simulink library "halout"  (R2021b)
settings: Solver=VariableStepAuto  StartTime=0.0  StopTime=10.0  RelTol=1e-3
undefined symbols (not defined in the file): C_TASK_5MS_S, FALSE, KHAL_CAN1TxReq_flg, KHAL_CAN2TxReq_flg, KHAL_CAN3FD3VCU1toNIDECTxReq_flg, KHAL_CAN3FD3VCU1TxReq_flg, KHAL_CAN3FD3VCU2E2E_flg, KHAL_CAN3FD3VCU2toNIDECE2E_flg, KHAL_CAN3FD3VCU2toNIDECTxReq_flg, KHAL_CAN3FD3VCU2TxReq_flg, KHAL_CAN3TxReq_flg, KHAL_CAN4FD4CE1000E2E_flg, KHAL_CAN4FD4CE1000TxReq_flg, KHAL_CAN4TxReq_flg, KHAL_CAN5TxReq_flg, KHAL_CAN7TxReq_flg, ONE_INT, TRUE, ZERO_INT
libraries: FVT_lib x258, simulink x115
(part 15 of 17)

== system halout/HAL_OUT/CAN4/FD4_CE100_0_0x116/HornCtrl ==
  HornCtrl : Inport
  Data Type Conversion : DataTypeConversion  OutDataTypeStr=uint8  RndMeth=Round
  CAN4_HornCtrl : Outport
  wires:
  Data Type Conversion/1 -> CAN4_HornCtrl/1
  HornCtrl/1 -> Data Type Conversion/1

== system halout/HAL_OUT/CAN4/FD4_CE100_0_0x116/LAPMWdwEnable ==
  LAPMWdwEnable : Inport
  Data Type Conversion : DataTypeConversion  OutDataTypeStr=uint8  RndMeth=Round
  CAN4_L_APM_WdwEnable : Outport
  wires:
  Data Type Conversion/1 -> CAN4_L_APM_WdwEnable/1
  LAPMWdwEnable/1 -> Data Type Conversion/1

== system halout/HAL_OUT/CAN4/FD4_CE100_0_0x116/LBSD ==
  LBSD : Inport
  Data Type Conversion : DataTypeConversion  OutDataTypeStr=uint8  RndMeth=Round
  CAN4_LBSD : Outport
  wires:
  Data Type Conversion/1 -> CAN4_LBSD/1
  LBSD/1 -> Data Type Conversion/1

== system halout/HAL_OUT/CAN4/FD4_CE100_0_0x116/LBeam ==
  LBeam : Inport
  Data Type Conversion : DataTypeConversion  OutDataTypeStr=uint8  RndMeth=Round
  CAN4_L_Beam : Outport
  wires:
  Data Type Conversion/1 -> CAN4_L_Beam/1
  LBeam/1 -> Data Type Conversion/1

== system halout/HAL_OUT/CAN4/FD4_CE100_0_0x116/LDRL ==
  LDRL : Inport
  Data Type Conversion : DataTypeConversion  OutDataTypeStr=uint8  RndMeth=Round
  CAN4_LDRL : Outport
  wires:
  Data Type Conversion/1 -> CAN4_LDRL/1
  LDRL/1 -> Data Type Conversion/1

== system halout/HAL_OUT/CAN4/FD4_CE100_0_0x116/LTurnLP ==
  LTurnLP : Inport
  Data Type Conversion : DataTypeConversion  OutDataTypeStr=uint8  RndMeth=Round
  CAN4_LTurnLP : Outport
  wires:
  Data Type Conversion/1 -> CAN4_LTurnLP/1
  LTurnLP/1 -> Data Type Conversion/1

== system halout/HAL_OUT/CAN4/FD4_CE100_0_0x116/LampPwr ==
  LampPwr : Inport
  Data Type Conversion : DataTypeConversion  OutDataTypeStr=uint8  RndMeth=Round
  CAN4_LampPwr : Outport
  wires:
  Data Type Conversion/1 -> CAN4_LampPwr/1
  LampPwr/1 -> Data Type Conversion/1

== system halout/HAL_OUT/CAN4/FD4_CE100_0_0x116/LockSetting ==
  LockSetting : Inport
  Data Type Conversion : DataTypeConversion  OutDataTypeStr=uint8  RndMeth=Round
  CAN4_LockSetting : Outport
  wires:
  Data Type Conversion/1 -> CAN4_LockSetting/1
  LockSetting/1 -> Data Type Conversion/1

== system halout/HAL_OUT/CAN4/FD4_CE100_0_0x116/MSACrlSta ==
  MSACrlSta : Inport
  Data Type Conversion : DataTypeConversion  OutDataTypeStr=uint8  RndMeth=Round
  CAN4_MSA_Crl_Sta : Outport
  wires:
  Data Type Conversion/1 -> CAN4_MSA_Crl_Sta/1
  MSACrlSta/1 -> Data Type Conversion/1

== system halout/HAL_OUT/CAN4/FD4_CE100_0_0x116/MirrorCtrl ==
  MirrorCtrl : Inport
  Data Type Conversion : DataTypeConversion  OutDataTypeStr=uint8  RndMeth=Round
  CAN4_MirrorCtrl : Outport
  wires:
  Data Type Conversion/1 -> CAN4_MirrorCtrl/1
  MirrorCtrl/1 -> Data Type Conversion/1

== system halout/HAL_OUT/CAN4/FD4_CE100_0_0x116/MirrorDefog ==
  MirrorDefog : Inport
  Data Type Conversion : DataTypeConversion  OutDataTypeStr=uint8  RndMeth=Round
  CAN4_MirrorDefog : Outport
  wires:
  Data Type Conversion/1 -> CAN4_MirrorDefog/1
  MirrorDefog/1 -> Data Type Conversion/1

== system halout/HAL_OUT/CAN4/FD4_CE100_0_0x116/PosLamp ==
  PosLamp : Inport
  Data Type Conversion : DataTypeConversion  OutDataTypeStr=uint8  RndMeth=Round
  CAN4_PosLamp : Outport
  wires:
  Data Type Conversion/1 -> CAN4_PosLamp/1
  PosLamp/1 -> Data Type Conversion/1

== system halout/HAL_OUT/CAN4/FD4_CE100_0_0x116/PsDoorSW ==
  PsDoorSW : Inport
  Data Type Conversion : DataTypeConversion  OutDataTypeStr=uint8  RndMeth=Round
  CAN4_PsDoorSW : Outport
  wires:
  Data Type Conversion/1 -> CAN4_PsDoorSW/1
  PsDoorSW/1 -> Data Type Conversion/1

== system halout/HAL_OUT/CAN4/FD4_CE100_0_0x116/PwrSta ==
  PwrSta : Inport
  Data Type Conversion : DataTypeConversion  OutDataTypeStr=uint8  RndMeth=Round
  CAN4_PwrSta : Outport
  wires:
  Data Type Conversion/1 -> CAN4_PwrSta/1
  PwrSta/1 -> Data Type Conversion/1

== system halout/HAL_OUT/CAN4/FD4_CE100_0_0x116/RBSD ==
  RBSD : Inport
  Data Type Conversion : DataTypeConversion  OutDataTypeStr=uint8  RndMeth=Round
  CAN4_RBSD : Outport
  wires:
  Data Type Conversion/1 -> CAN4_RBSD/1
  RBSD/1 -> Data Type Conversion/1

== system halout/HAL_OUT/CAN4/FD4_CE100_0_0x116/RCVCU1CAN4 ==
  RCVCU1CAN4 : Inport
  Data Type Conversion : DataTypeConversion  OutDataTypeStr=uint8  RndMeth=Round
  CAN4_RC_VCU1_CAN4 : Outport
  wires:
  Data Type Conversion/1 -> CAN4_RC_VCU1_CAN4/1
  RCVCU1CAN4/1 -> Data Type Conversion/1

== system halout/HAL_OUT/CAN4/FD4_CE100_0_0x116/RDRL ==
  RDRL : Inport
  Data Type Conversion : DataTypeConversion  OutDataTypeStr=uint8  RndMeth=Round
  CAN4_RDRL : Outport
  wires:
  Data Type Conversion/1 -> CAN4_RDRL/1
  RDRL/1 -> Data Type Conversion/1

== system halout/HAL_OUT/CAN4/FD4_CE100_0_0x116/RLDoorSW ==
  RLDoorSW : Inport
  Data Type Conversion : DataTypeConversion  OutDataTypeStr=uint8  RndMeth=Round
  CAN4_RLDoorSW : Outport
  wires:
  Data Type Conversion/1 -> CAN4_RLDoorSW/1
  RLDoorSW/1 -> Data Type Conversion/1

== system halout/HAL_OUT/CAN4/FD4_CE100_0_0x116/RRDoorSW ==
  RRDoorSW : Inport
  Data Type Conversion : DataTypeConversion  OutDataTypeStr=uint8  RndMeth=Round
  CAN4_RRDoorSW : Outport
  wires:
  Data Type Conversion/1 -> CAN4_RRDoorSW/1
  RRDoorSW/1 -> Data Type Conversion/1

== system halout/HAL_OUT/CAN4/FD4_CE100_0_0x116/RTurnLP ==
  RTurnLP : Inport
  Data Type Conversion : DataTypeConversion  OutDataTypeStr=uint8  RndMeth=Round
  CAN4_RTurnLP : Outport
  wires:
  Data Type Conversion/1 -> CAN4_RTurnLP/1
  RTurnLP/1 -> Data Type Conversion/1

== system halout/HAL_OUT/CAN4/FD4_CE100_0_0x116/ReBrakeLPReq ==
  ReBrakeLPReq : Inport
  Data Type Conversion : DataTypeConversion  OutDataTypeStr=uint8  RndMeth=Round
  CAN4_ReBrakeLPReq : Outport
  wires:
  Data Type Conversion/1 -> CAN4_ReBrakeLPReq/1
  ReBrakeLPReq/1 -> Data Type Conversion/1

== system halout/HAL_OUT/CAN4/FD4_CE100_0_0x116/ReverseLamp ==
  ReverseLamp : Inport
  Data Type Conversion : DataTypeConversion  OutDataTypeStr=uint8  RndMeth=Round
  CAN4_ReverseLamp : Outport
  wires:
  Data Type Conversion/1 -> CAN4_ReverseLamp/1
  ReverseLamp/1 -> Data Type Conversion/1

== system halout/HAL_OUT/CAN4/FD4_CE100_0_0x116/RoomLampH ==
  RoomLampH : Inport
  Data Type Conversion : DataTypeConversion  OutDataTypeStr=uint8  RndMeth=Round
  CAN4_RoomLampH : Outport
  wires:
  Data Type Conversion/1 -> CAN4_RoomLampH/1
  RoomLampH/1 -> Data Type Conversion/1

== system halout/HAL_OUT/CAN4/FD4_CE100_0_0x116/RoomLampL ==
  RoomLampL : Inport
  Data Type Conversion : DataTypeConversion  OutDataTypeStr=uint8  RndMeth=Round
  CAN4_RoomLampL : Outport
  wires:
  Data Type Conversion/1 -> CAN4_RoomLampL/1
  RoomLampL/1 -> Data Type Conversion/1

== system halout/HAL_OUT/CAN4/FD4_CE100_0_0x116/RrChargingDoorCtrl ==
  RrChargingDoorCtrl : Inport
  Data Type Conversion : DataTypeConversion  OutDataTypeStr=uint8  RndMeth=Round
  CAN4_Rr_ChargingDoorCtrl : Outport
  wires:
  Data Type Conversion/1 -> CAN4_Rr_ChargingDoorCtrl/1
  RrChargingDoorCtrl/1 -> Data Type Conversion/1

== system halout/HAL_OUT/CAN4/FD4_CE100_0_0x116/RrDefog ==
  RrDefog : Inport
  Data Type Conversion : DataTypeConversion  OutDataTypeStr=uint8  RndMeth=Round
  CAN4_Rr_Defog : Outport
  wires:
  Data Type Conversion/1 -> CAN4_Rr_Defog/1
  RrDefog/1 -> Data Type Conversion/1

== system halout/HAL_OUT/CAN4/FD4_CE100_0_0x116/RrFogLamp ==
  RrFogLamp : Inport
  Data Type Conversion : DataTypeConversion  OutDataTypeStr=uint8  RndMeth=Round
  CAN4_Rr_FogLamp : Outport
  wires:
  Data Type Conversion/1 -> CAN4_Rr_FogLamp/1
  RrFogLamp/1 -> Data Type Conversion/1

== system halout/HAL_OUT/CAN4/FD4_CE100_0_0x116/RrWiper ==
  RrWiper : Inport
  Data Type Conversion : DataTypeConversion  OutDataTypeStr=uint8  RndMeth=Round
  CAN4_Rr_Wiper : Outport
  wires:
  Data Type Conversion/1 -> CAN4_Rr_Wiper/1
  RrWiper/1 -> Data Type Conversion/1

== system halout/HAL_OUT/CAN4/FD4_CE100_0_0x116/ShiftGearPosn ==
  ShiftGearPosn : Inport
  Data Type Conversion : DataTypeConversion  OutDataTypeStr=uint8  RndMeth=Round
  CAN4_ShiftGearPosn : Outport
  wires:
  Data Type Conversion/1 -> CAN4_ShiftGearPosn/1
  ShiftGearPosn/1 -> Data Type Conversion/1

== system halout/HAL_OUT/CAN4/FD4_CE100_0_0x116/TailgateHDSW ==
  TailgateHDSW : Inport
  Data Type Conversion : DataTypeConversion  OutDataTypeStr=uint8  RndMeth=Round
  CAN4_TailgateHDSW : Outport
  wires:
  Data Type Conversion/1 -> CAN4_TailgateHDSW/1
  TailgateHDSW/1 -> Data Type Conversion/1

== system halout/HAL_OUT/CAN4/FD4_CE100_0_0x116/TailgateRemote ==
  TailgateRemote : Inport
  Data Type Conversion : DataTypeConversion  OutDataTypeStr=uint8  RndMeth=Round
  CAN4_TailgateRemote : Outport
  wires:
  Data Type Conversion/1 -> CAN4_TailgateRemote/1
  TailgateRemote/1 -> Data Type Conversion/1

== system halout/HAL_OUT/CAN4/FD4_CE100_0_0x116/TailgateSW ==
  TailgateSW : Inport
  Data Type Conversion : DataTypeConversion  OutDataTypeStr=uint8  RndMeth=Round
  CAN4_Tailgate_SW : Outport
  wires:
  Data Type Conversion/1 -> CAN4_Tailgate_SW/1
  TailgateSW/1 -> Data Type Conversion/1

== system halout/HAL_OUT/CAN4/FD4_CE100_0_0x116/TimeSNDKCFbk ==
  TimeSNDKCFbk : Inport
  Data Type Conversion : DataTypeConversion  OutDataTypeStr=uint32  RndMeth=Round
  CAN4_TimeSNDKCFbk : Outport
  wires:
  Data Type Conversion/1 -> CAN4_TimeSNDKCFbk/1
  TimeSNDKCFbk/1 -> Data Type Conversion/1

== system halout/HAL_OUT/CAN4/FD4_CE100_0_0x116/TrunkRel ==
  TrunkRel : Inport
  Data Type Conversion : DataTypeConversion  OutDataTypeStr=uint8  RndMeth=Round
  CAN4_TrunkRel : Outport
  wires:
  Data Type Conversion/1 -> CAN4_TrunkRel/1
  TrunkRel/1 -> Data Type Conversion/1

== system halout/HAL_OUT/CAN4/FD4_CE100_0_0x116/WasherCtrl ==
  WasherCtrl : Inport
  Data Type Conversion : DataTypeConversion  OutDataTypeStr=uint8  RndMeth=Round
  CAN4_WasherCtrl : Outport
  wires:
  Data Type Conversion/1 -> CAN4_WasherCtrl/1
  WasherCtrl/1 -> Data Type Conversion/1

== system halout/HAL_OUT/CAN4/FD4_CE100_0_0x116/WiperFixMode ==
  WiperFixMode : Inport
  Data Type Conversion : DataTypeConversion  OutDataTypeStr=uint8  RndMeth=Round
  CAN4_WiperFixMode : Outport
  wires:
  Data Type Conversion/1 -> CAN4_WiperFixMode/1
  WiperFixMode/1 -> Data Type Conversion/1

== system halout/HAL_OUT/CAN4/FD4_CE100_1_0x182/ACSubMode ==
  ACSubMode : Inport
  Data Type Conversion : DataTypeConversion  OutDataTypeStr=uint8  RndMeth=Round
  CAN4_ACSubMode : Outport
  wires:
  Data Type Conversion/1 -> CAN4_ACSubMode/1
  ACSubMode/1 -> Data Type Conversion/1

== system halout/HAL_OUT/CAN4/FD4_CE100_1_0x182/APTCActFrRiPwr ==
  APTCActFrRiPwr : Inport
  Data Type Conversion : DataTypeConversion  OutDataTypeStr=uint8  RndMeth=Round
  convert_out : FVT_lib/hal/convert_out  gain=25  offset=0
  CAN4_APTC_ActFrRiPwr : Outport
  wires:
  Data Type Conversion/1 -> CAN4_APTC_ActFrRiPwr/1
  convert_out/1 -> Data Type Conversion/1
  APTCActFrRiPwr/1 -> convert_out/1

== system halout/HAL_OUT/CAN4/FD4_CE100_1_0x182/BatLoopActWtFlw ==
  BatLoopActWtFlw : Inport
  Data Type Conversion : DataTypeConversion  OutDataTypeStr=uint8  RndMeth=Round
  convert_out : FVT_lib/hal/convert_out  gain=0.1  offset=-5
  CAN4_BatLoopActWtFlw : Outport
  wires:
  Data Type Conversion/1 -> CAN4_BatLoopActWtFlw/1
  convert_out/1 -> Data Type Conversion/1
  BatLoopActWtFlw/1 -> convert_out/1

== system halout/HAL_OUT/CAN4/FD4_CE100_1_0x182/BatteryMode ==
  BatteryMode : Inport
  Data Type Conversion : DataTypeConversion  OutDataTypeStr=uint8  RndMeth=Round
  CAN4_BatteryMode : Outport
  wires:
  Data Type Conversion/1 -> CAN4_BatteryMode/1
  BatteryMode/1 -> Data Type Conversion/1

== system halout/HAL_OUT/CAN4/FD4_CE100_1_0x182/CCUACLampSts ==
  CCUACLampSts : Inport
  Data Type Conversion : DataTypeConversion  OutDataTypeStr=uint8  RndMeth=Round
  CAN4_CCU_ACLampSts : Outport
  wires:
  Data Type Conversion/1 -> CAN4_CCU_ACLampSts/1
  CCUACLampSts/1 -> Data Type Conversion/1

== system halout/HAL_OUT/CAN4/FD4_CE100_1_0x182/CCUACMaxLampSts ==
  CCUACMaxLampSts : Inport
  Data Type Conversion : DataTypeConversion  OutDataTypeStr=uint8  RndMeth=Round
  CAN4_CCU_ACMaxLampSts : Outport
  wires:
  Data Type Conversion/1 -> CAN4_CCU_ACMaxLampSts/1
  CCUACMaxLampSts/1 -> Data Type Conversion/1

== system halout/HAL_OUT/CAN4/FD4_CE100_1_0x182/CCUAutoLampSts ==
  CCUAutoLampSts : Inport
  Data Type Conversion : DataTypeConversion  OutDataTypeStr=uint8  RndMeth=Round
  CAN4_CCU_AutoLampSts : Outport
  wires:
  Data Type Conversion/1 -> CAN4_CCU_AutoLampSts/1
  CCUAutoLampSts/1 -> Data Type Conversion/1

== system halout/HAL_OUT/CAN4/FD4_CE100_1_0x182/CCUAutoMidLampSts ==
  CCUAutoMidLampSts : Inport
  Data Type Conversion : DataTypeConversion  OutDataTypeStr=uint8  RndMeth=Round
  CAN4_CCU_AutoMidLampSts : Outport
  wires:
  Data Type Conversion/1 -> CAN4_CCU_AutoMidLampSts/1
  CCUAutoMidLampSts/1 -> Data Type Conversion/1

== system halout/HAL_OUT/CAN4/FD4_CE100_1_0x182/CCUCbnPreACWkSts ==
  CCUCbnPreACWkSts : Inport
  Data Type Conversion : DataTypeConversion  OutDataTypeStr=uint8  RndMeth=Round
  CAN4_CCU_CbnPreACWkSts : Outport
  wires:
  Data Type Conversion/1 -> CAN4_CCU_CbnPreACWkSts/1
  CCUCbnPreACWkSts/1 -> Data Type Conversion/1

== system halout/HAL_OUT/CAN4/FD4_CE100_1_0x182/CCUCbnPreEstimdTi ==
  CCUCbnPreEstimdTi : Inport
  Data Type Conversion : DataTypeConversion  OutDataTypeStr=uint8  RndMeth=Round
  CAN4_CCU_CbnPreEstimdTi : Outport
  wires:
  Data Type Conversion/1 -> CAN4_CCU_CbnPreEstimdTi/1
  CCUCbnPreEstimdTi/1 -> Data Type Conversion/1

== system halout/HAL_OUT/CAN4/FD4_CE100_1_0x182/CCUCbnPreSts ==
  CCUCbnPreSts : Inport
  Data Type Conversion : DataTypeConversion  OutDataTypeStr=uint8  RndMeth=Round
  CAN4_CCU_CbnPreSts : Outport
  wires:
  Data Type Conversion/1 -> CAN4_CCU_CbnPreSts/1
  CCUCbnPreSts/1 -> Data Type Conversion/1

== system halout/HAL_OUT/CAN4/FD4_CE100_1_0x182/CCUDispalyRequest ==
  CCUDispalyRequest : Inport
  Data Type Conversion : DataTypeConversion  OutDataTypeStr=uint8  RndMeth=Round
  CAN4_CCU_Dispaly_Request : Outport
  wires:
  Data Type Conversion/1 -> CAN4_CCU_Dispaly_Request/1
  CCUDispalyRequest/1 -> Data Type Conversion/1

== system halout/HAL_OUT/CAN4/FD4_CE100_1_0x182/CCUEcoSts ==
  CCUEcoSts : Inport
  Data Type Conversion : DataTypeConversion  OutDataTypeStr=uint8  RndMeth=Round
  CAN4_CCU_EcoSts : Outport
  wires:
  Data Type Conversion/1 -> CAN4_CCU_EcoSts/1
  CCUEcoSts/1 -> Data Type Conversion/1

== system halout/HAL_OUT/CAN4/FD4_CE100_1_0x182/CCUFrtOnOffLampSts ==
  CCUFrtOnOffLampSts : Inport
  Data Type Conversion : DataTypeConversion  OutDataTypeStr=uint8  RndMeth=Round
  CAN4_CCU_FrtOnOffLampSts : Outport
  wires:
  Data Type Conversion/1 -> CAN4_CCU_FrtOnOffLampSts/1
  CCUFrtOnOffLampSts/1 -> Data Type Conversion/1

== system halout/HAL_OUT/CAN4/FD4_CE100_1_0x182/CCUHEATMaxLampSts ==
  CCUHEATMaxLampSts : Inport
  Data Type Conversion : DataTypeConversion  OutDataTypeStr=uint8  RndMeth=Round
  CAN4_CCU_HEATMaxLampSts : Outport
  wires:
  Data Type Conversion/1 -> CAN4_CCU_HEATMaxLampSts/1
  CCUHEATMaxLampSts/1 -> Data Type Conversion/1

== system halout/HAL_OUT/CAN4/FD4_CE100_1_0x182/CCUHiVoltageReq ==
  CCUHiVoltageReq : Inport
  Data Type Conversion : DataTypeConversion  OutDataTypeStr=uint8  RndMeth=Round
  CAN4_CCU_HiVoltageReq : Outport
  wires:
  Data Type Conversion/1 -> CAN4_CCU_HiVoltageReq/1
  CCUHiVoltageReq/1 -> Data Type Conversion/1

== system halout/HAL_OUT/CAN4/FD4_CE100_1_0x182/CCURrOnOffLampSts ==
  CCURrOnOffLampSts : Inport
  Data Type Conversion : DataTypeConversion  OutDataTypeStr=uint8  RndMeth=Round
  CAN4_CCU_RrOnOffLampSts : Outport
  wires:
  Data Type Conversion/1 -> CAN4_CCU_RrOnOffLampSts/1
  CCURrOnOffLampSts/1 -> Data Type Conversion/1

== system halout/HAL_OUT/CAN4/FD4_CE100_1_0x182/CCUSyncLampSts ==
  CCUSyncLampSts : Inport
  Data Type Conversion : DataTypeConversion  OutDataTypeStr=uint8  RndMeth=Round
  CAN4_CCU_SyncLampSts : Outport
  wires:
  Data Type Conversion/1 -> CAN4_CCU_SyncLampSts/1
  CCUSyncLampSts/1 -> Data Type Conversion/1

== system halout/HAL_OUT/CAN4/FD4_CE100_1_0x182/CabinMode ==
  CabinMode : Inport
  Data Type Conversion : DataTypeConversion  OutDataTypeStr=uint8  RndMeth=Round
  CAN4_CabinMode : Outport
  wires:
  Data Type Conversion/1 -> CAN4_CabinMode/1
  CabinMode/1 -> Data Type Conversion/1

== system halout/HAL_OUT/CAN4/FD4_CE100_1_0x182/CoolgFanActDuty ==
  CoolgFanActDuty : Inport
  Data Type Conversion : DataTypeConversion  OutDataTypeStr=uint8  RndMeth=Round
  convert_out : FVT_lib/hal/convert_out  gain=0.5  offset=0
  CAN4_CoolgFanActDuty : Outport
  wires:
  Data Type Conversion/1 -> CAN4_CoolgFanActDuty/1
  convert_out/1 -> Data Type Conversion/1
  CoolgFanActDuty/1 -> convert_out/1

== system halout/HAL_OUT/CAN4/FD4_CE100_1_0x182/DeiceModReq ==
  DeiceModReq : Inport
  Data Type Conversion : DataTypeConversion  OutDataTypeStr=uint8  RndMeth=Round
  CAN4_DeiceModReq : Outport
  wires:
  Data Type Conversion/1 -> CAN4_DeiceModReq/1
  DeiceModReq/1 -> Data Type Conversion/1

== system halout/HAL_OUT/CAN4/FD4_CE100_1_0x182/EDriveMode ==
  EDriveMode : Inport
  Data Type Conversion : DataTypeConversion  OutDataTypeStr=uint8  RndMeth=Round
  CAN4_EDriveMode : Outport
  wires:
  Data Type Conversion/1 -> CAN4_EDriveMode/1
  EDriveMode/1 -> Data Type Conversion/1

== system halout/HAL_OUT/CAN4/FD4_CE100_1_0x182/FDBlowerCmd ==
  FDBlowerCmd : Inport
  Data Type Conversion : DataTypeConversion  OutDataTypeStr=uint8  RndMeth=Round
  convert_out : FVT_lib/hal/convert_out  gain=0.8  offset=0
  CAN4_FD_Blower_Cmd : Outport
  wires:
  Data Type Conversion/1 -> CAN4_FD_Blower_Cmd/1
  convert_out/1 -> Data Type Conversion/1
  FDBlowerCmd/1 -> convert_out/1

== system halout/HAL_OUT/CAN4/FD4_CE100_1_0x182/FDCTHCMCLEVentYSta ==
  FDCTHCMCLEVentYSta : Inport
  Data Type Conversion : DataTypeConversion  OutDataTypeStr=uint8  RndMeth=Round
  CAN4_FDC_THCM_CLEVentY_Sta : Outport
  wires:
  Data Type Conversion/1 -> CAN4_FDC_THCM_CLEVentY_Sta/1
  FDCTHCMCLEVentYSta/1 -> Data Type Conversion/1

== system halout/HAL_OUT/CAN4/FD4_CE100_1_0x182/FDCTHCMCLEVentZSta ==
  FDCTHCMCLEVentZSta : Inport
  Data Type Conversion : DataTypeConversion  OutDataTypeStr=uint8  RndMeth=Round
  CAN4_FDC_THCM_CLEVentZ_Sta : Outport
  wires:
  Data Type Conversion/1 -> CAN4_FDC_THCM_CLEVentZ_Sta/1
  FDCTHCMCLEVentZSta/1 -> Data Type Conversion/1

== system halout/HAL_OUT/CAN4/FD4_CE100_1_0x182/FDCTHCMCLVentSta ==
  FDCTHCMCLVentSta : Inport
  Data Type Conversion : DataTypeConversion  OutDataTypeStr=uint8  RndMeth=Round
  CAN4_FDC_THCM_CLVent_Sta : Outport
  wires:
  Data Type Conversion/1 -> CAN4_FDC_THCM_CLVent_Sta/1
  FDCTHCMCLVentSta/1 -> Data Type Conversion/1

== system halout/HAL_OUT/CAN4/FD4_CE100_1_0x182/FDCTHCMCREVentYSta ==
  FDCTHCMCREVentYSta : Inport
  Data Type Conversion : DataTypeConversion  OutDataTypeStr=uint8  RndMeth=Round
  CAN4_FDC_THCM_CREVentY_Sta : Outport
  wires:
  Data Type Conversion/1 -> CAN4_FDC_THCM_CREVentY_Sta/1
  FDCTHCMCREVentYSta/1 -> Data Type Conversion/1

== system halout/HAL_OUT/CAN4/FD4_CE100_1_0x182/FDCTHCMCREVentZSta ==
  FDCTHCMCREVentZSta : Inport
  Data Type Conversion : DataTypeConversion  OutDataTypeStr=uint8  RndMeth=Round
  CAN4_FDC_THCM_CREVentZ_Sta : Outport
  wires:
  Data Type Conversion/1 -> CAN4_FDC_THCM_CREVentZ_Sta/1
  FDCTHCMCREVentZSta/1 -> Data Type Conversion/1

== system halout/HAL_OUT/CAN4/FD4_CE100_1_0x182/FDCTHCMCRVentSta ==
  FDCTHCMCRVentSta : Inport
  Data Type Conversion : DataTypeConversion  OutDataTypeStr=uint8  RndMeth=Round
  CAN4_FDC_THCM_CRVent_Sta : Outport
  wires:
  Data Type Conversion/1 -> CAN4_FDC_THCM_CRVent_Sta/1
  FDCTHCMCRVentSta/1 -> Data Type Conversion/1

== system halout/HAL_OUT/CAN4/FD4_CE100_1_0x182/FDCTHCMDrEVentModeSta ==
  FDCTHCMDrEVentModeSta : Inport
  Data Type Conversion : DataTypeConversion  OutDataTypeStr=uint8  RndMeth=Round
  CAN4_FDC_THCM_DrEVentMode_Sta : Outport
  wires:
  Data Type Conversion/1 -> CAN4_FDC_THCM_DrEVentMode_Sta/1
  FDCTHCMDrEVentModeSta/1 -> Data Type Conversion/1

== system halout/HAL_OUT/CAN4/FD4_CE100_1_0x182/FDCTHCMDrEVentYSta ==
  FDCTHCMDrEVentYSta : Inport
  Data Type Conversion : DataTypeConversion  OutDataTypeStr=uint8  RndMeth=Round
  CAN4_FDC_THCM_DrEVentY_Sta : Outport
  wires:
  Data Type Conversion/1 -> CAN4_FDC_THCM_DrEVentY_Sta/1
  FDCTHCMDrEVentYSta/1 -> Data Type Conversion/1

== system halout/HAL_OUT/CAN4/FD4_CE100_1_0x182/FDCTHCMDrEVentZSta ==
  FDCTHCMDrEVentZSta : Inport
  Data Type Conversion : DataTypeConversion  OutDataTypeStr=uint8  RndMeth=Round
  CAN4_FDC_THCM_DrEVentZ_Sta : Outport
  wires:
  Data Type Conversion/1 -> CAN4_FDC_THCM_DrEVentZ_Sta/1
  FDCTHCMDrEVentZSta/1 -> Data Type Conversion/1

== system halout/HAL_OUT/CAN4/FD4_CE100_1_0x182/FDCTHCMDrVentSta ==
  FDCTHCMDrVentSta : Inport
  Data Type Conversion : DataTypeConversion  OutDataTypeStr=uint8  RndMeth=Round
  CAN4_FDC_THCM_DrVent_Sta : Outport
  wires:
  Data Type Conversion/1 -> CAN4_FDC_THCM_DrVent_Sta/1
  FDCTHCMDrVentSta/1 -> Data Type Conversion/1

== system halout/HAL_OUT/CAN4/FD4_CE100_1_0x182/FDCTHCMPsEVentModeSta ==
  FDCTHCMPsEVentModeSta : Inport
  Data Type Conversion : DataTypeConversion  OutDataTypeStr=uint8  RndMeth=Round
  CAN4_FDC_THCM_PsEVentMode_Sta : Outport
  wires:
  Data Type Conversion/1 -> CAN4_FDC_THCM_PsEVentMode_Sta/1
  FDCTHCMPsEVentModeSta/1 -> Data Type Conversion/1

== system halout/HAL_OUT/CAN4/FD4_CE100_1_0x182/FDCTHCMPsEVentYSta ==
  FDCTHCMPsEVentYSta : Inport
  Data Type Conversion : DataTypeConversion  OutDataTypeStr=uint8  RndMeth=Round
  CAN4_FDC_THCM_PsEVentY_Sta : Outport
  wires:
  Data Type Conversion/1 -> CAN4_FDC_THCM_PsEVentY_Sta/1
  FDCTHCMPsEVentYSta/1 -> Data Type Conversion/1

== system halout/HAL_OUT/CAN4/FD4_CE100_1_0x182/FDCTHCMPsEVentZSta ==
  FDCTHCMPsEVentZSta : Inport
  Data Type Conversion : DataTypeConversion  OutDataTypeStr=uint8  RndMeth=Round
  CAN4_FDC_THCM_PsEVentZ_Sta : Outport
  wires:
  Data Type Conversion/1 -> CAN4_FDC_THCM_PsEVentZ_Sta/1
  FDCTHCMPsEVentZSta/1 -> Data Type Conversion/1

== system halout/HAL_OUT/CAN4/FD4_CE100_1_0x182/FDCTHCMPsVentSta ==
  FDCTHCMPsVentSta : Inport
  Data Type Conversion : DataTypeConversion  OutDataTypeStr=uint8  RndMeth=Round
  CAN4_FDC_THCM_PsVent_Sta : Outport
  wires:
  Data Type Conversion/1 -> CAN4_FDC_THCM_PsVent_Sta/1
  FDCTHCMPsVentSta/1 -> Data Type Conversion/1

== system halout/HAL_OUT/CAN4/FD4_CE100_1_0x182/FDCompCmd ==
  FDCompCmd : Inport
  Data Type Conversion : DataTypeConversion  OutDataTypeStr=uint16  RndMeth=Round
  convert_out : FVT_lib/hal/convert_out  gain=0.5  offset=0
  CAN4_FD_Comp_Cmd : Outport
  wires:
  Data Type Conversion/1 -> CAN4_FD_Comp_Cmd/1
  convert_out/1 -> Data Type Conversion/1
  FDCompCmd/1 -> convert_out/1

== system halout/HAL_OUT/CAN4/FD4_CE100_1_0x182/FDEWP1Cmd ==
  FDEWP1Cmd : Inport
  Data Type Conversion : DataTypeConversion  OutDataTypeStr=uint8  RndMeth=Round
  CAN4_FD_EWP1_Cmd : Outport
  wires:
  Data Type Conversion/1 -> CAN4_FD_EWP1_Cmd/1
  FDEWP1Cmd/1 -> Data Type Conversion/1

== system halout/HAL_OUT/CAN4/FD4_CE100_1_0x182/FDEWP2Cmd ==
  FDEWP2Cmd : Inport
  Data Type Conversion : DataTypeConversion  OutDataTypeStr=uint8  RndMeth=Round
  CAN4_FD_EWP2_Cmd : Outport
  wires:
  Data Type Conversion/1 -> CAN4_FD_EWP2_Cmd/1
  FDEWP2Cmd/1 -> Data Type Conversion/1

== system halout/HAL_OUT/CAN4/FD4_CE100_1_0x182/FDEWP3Cmd ==
  FDEWP3Cmd : Inport
  Data Type Conversion : DataTypeConversion  OutDataTypeStr=uint8  RndMeth=Round
  CAN4_FD_EWP3_Cmd : Outport
  wires:
  Data Type Conversion/1 -> CAN4_FD_EWP3_Cmd/1
  FDEWP3Cmd/1 -> Data Type Conversion/1

== system halout/HAL_OUT/CAN4/FD4_CE100_1_0x182/FDEXV1Cmd ==
  FDEXV1Cmd : Inport
  Data Type Conversion : DataTypeConversion  OutDataTypeStr=uint16  RndMeth=Round
  CAN4_FD_EXV1_Cmd : Outport
  wires:
  Data Type Conversion/1 -> CAN4_FD_EXV1_Cmd/1
  FDEXV1Cmd/1 -> Data Type Conversion/1

== system halout/HAL_OUT/CAN4/FD4_CE100_1_0x182/FDEXV2Cmd ==
  FDEXV2Cmd : Inport
  Data Type Conversion : DataTypeConversion  OutDataTypeStr=uint16  RndMeth=Round
  CAN4_FD_EXV2_Cmd : Outport
  wires:
  Data Type Conversion/1 -> CAN4_FD_EXV2_Cmd/1
  FDEXV2Cmd/1 -> Data Type Conversion/1

== system halout/HAL_OUT/CAN4/FD4_CE100_1_0x182/FDFWVCmd ==
  FDFWVCmd : Inport
  Data Type Conversion : DataTypeConversion  OutDataTypeStr=uint8  RndMeth=Round
  CAN4_FD_FWV_Cmd : Outport
  wires:
  Data Type Conversion/1 -> CAN4_FD_FWV_Cmd/1
  FDFWVCmd/1 -> Data Type Conversion/1

== system halout/HAL_OUT/CAN4/FD4_CE100_1_0x182/FDFrLeAPTCHeatPwrCmd ==
  FDFrLeAPTCHeatPwrCmd : Inport
  Data Type Conversion : DataTypeConversion  OutDataTypeStr=uint8  RndMeth=Round
  convert_out : FVT_lib/hal/convert_out  gain=25  offset=0
  CAN4_FD_FrLeAPTCHeatPwr_Cmd : Outport
  wires:
  Data Type Conversion/1 -> CAN4_FD_FrLeAPTCHeatPwr_Cmd/1
  convert_out/1 -> Data Type Conversion/1
  FDFrLeAPTCHeatPwrCmd/1 -> convert_out/1

== system halout/HAL_OUT/CAN4/FD4_CE100_1_0x182/FDFrRiAPTCHeatPwrCmd ==
  FDFrRiAPTCHeatPwrCmd : Inport
  Data Type Conversion : DataTypeConversion  OutDataTypeStr=uint8  RndMeth=Round
  convert_out : FVT_lib/hal/convert_out  gain=25  offset=0
  CAN4_FD_FrRiAPTCHeatPwr_Cmd : Outport
  wires:
  Data Type Conversion/1 -> CAN4_FD_FrRiAPTCHeatPwr_Cmd/1
  convert_out/1 -> Data Type Conversion/1
  FDFrRiAPTCHeatPwrCmd/1 -> convert_out/1

== system halout/HAL_OUT/CAN4/FD4_CE100_1_0x182/FDFrWPTCHeatPwrCmd ==
  FDFrWPTCHeatPwrCmd : Inport
  Data Type Conversion : DataTypeConversion  OutDataTypeStr=uint16  RndMeth=Round
  CAN4_FD_FrWPTCHeatPwr_Cmd : Outport
  wires:
  Data Type Conversion/1 -> CAN4_FD_FrWPTCHeatPwr_Cmd/1
  FDFrWPTCHeatPwrCmd/1 -> Data Type Conversion/1

== system halout/HAL_OUT/CAN4/FD4_CE100_1_0x182/FDRecyAutoCmd ==
  FDRecyAutoCmd : Inport
  Data Type Conversion : DataTypeConversion  OutDataTypeStr=uint8  RndMeth=Round
  CAN4_FD_RecyAuto_Cmd : Outport
  wires:
  Data Type Conversion/1 -> CAN4_FD_RecyAuto_Cmd/1
  FDRecyAutoCmd/1 -> Data Type Conversion/1

== system halout/HAL_OUT/CAN4/FD4_CE100_1_0x182/FDRrAPTCHeatPwrCmd ==
  FDRrAPTCHeatPwrCmd : Inport
  Data Type Conversion : DataTypeConversion  OutDataTypeStr=uint8  RndMeth=Round
  convert_out : FVT_lib/hal/convert_out  gain=25  offset=0
  CAN4_FD_RrAPTCHeatPwr_Cmd : Outport
  wires:
  Data Type Conversion/1 -> CAN4_FD_RrAPTCHeatPwr_Cmd/1
  convert_out/1 -> Data Type Conversion/1
  FDRrAPTCHeatPwrCmd/1 -> convert_out/1

== system halout/HAL_OUT/CAN4/FD4_CE100_1_0x182/FDSOTXVCmd ==
  FDSOTXVCmd : Inport
  Data Type Conversion : DataTypeConversion  OutDataTypeStr=uint8  RndMeth=Round
  CAN4_FD_SOTXV_Cmd : Outport
  wires:
  Data Type Conversion/1 -> CAN4_FD_SOTXV_Cmd/1
  FDSOTXVCmd/1 -> Data Type Conversion/1

== system halout/HAL_OUT/CAN4/FD4_CE100_1_0x182/FDSOV1Cmd ==
  FDSOV1Cmd : Inport
  Data Type Conversion : DataTypeConversion  OutDataTypeStr=uint8  RndMeth=Round
  CAN4_FD_SOV1_Cmd : Outport
  wires:
  Data Type Conversion/1 -> CAN4_FD_SOV1_Cmd/1
  FDSOV1Cmd/1 -> Data Type Conversion/1

== system halout/HAL_OUT/CAN4/FD4_CE100_1_0x182/FDSOV2Cmd ==
  FDSOV2Cmd : Inport
  Data Type Conversion : DataTypeConversion  OutDataTypeStr=uint8  RndMeth=Round
  CAN4_FD_SOV2_Cmd : Outport
  wires:
  Data Type Conversion/1 -> CAN4_FD_SOV2_Cmd/1
  FDSOV2Cmd/1 -> Data Type Conversion/1

== system halout/HAL_OUT/CAN4/FD4_CE100_1_0x182/FDSOV3Cmd ==
  FDSOV3Cmd : Inport
  Data Type Conversion : DataTypeConversion  OutDataTypeStr=uint8  RndMeth=Round
  CAN4_FD_SOV3_Cmd : Outport
  wires:
  Data Type Conversion/1 -> CAN4_FD_SOV3_Cmd/1
  FDSOV3Cmd/1 -> Data Type Conversion/1

== system halout/HAL_OUT/CAN4/FD4_CE100_1_0x182/FDTWVCmd ==
  FDTWVCmd : Inport
  Data Type Conversion : DataTypeConversion  OutDataTypeStr=uint8  RndMeth=Round
  convert_out : FVT_lib/hal/convert_out  gain=0.392  offset=0
  CAN4_FD_TWV_Cmd : Outport
  wires:
  Data Type Conversion/1 -> CAN4_FD_TWV_Cmd/1
  convert_out/1 -> Data Type Conversion/1
  FDTWVCmd/1 -> convert_out/1

== system halout/HAL_OUT/CAN4/FD4_CE100_1_0x182/FrCoolantflow ==
  FrCoolantflow : Inport
  Data Type Conversion : DataTypeConversion  OutDataTypeStr=uint8  RndMeth=Round
  convert_out : FVT_lib/hal/convert_out  gain=0.25  offset=0
  CAN4_Fr_Coolantflow : Outport
  wires:
  Data Type Conversion/1 -> CAN4_Fr_Coolantflow/1
  convert_out/1 -> Data Type Conversion/1
  FrCoolantflow/1 -> convert_out/1

== system halout/HAL_OUT/CAN4/FD4_CE100_1_0x182/FrCoolanttemp ==
  FrCoolanttemp : Inport
  Data Type Conversion : DataTypeConversion  OutDataTypeStr=uint16  RndMeth=Round
  convert_out : FVT_lib/hal/convert_out  gain=1  offset=-40
  CAN4_Fr_Coolanttemp : Outport
  wires:
  Data Type Conversion/1 -> CAN4_Fr_Coolanttemp/1
  convert_out/1 -> Data Type Conversion/1
  FrCoolanttemp/1 -> convert_out/1

== system halout/HAL_OUT/CAN4/FD4_CE100_1_0x182/HPThermalRecoveryReq ==
  HPThermalRecoveryReq : Inport
  Data Type Conversion : DataTypeConversion  OutDataTypeStr=uint8  RndMeth=Round
  CAN4_HPThermalRecoveryReq : Outport
  wires:
  Data Type Conversion/1 -> CAN4_HPThermalRecoveryReq/1
  HPThermalRecoveryReq/1 -> Data Type Conversion/1

== system halout/HAL_OUT/CAN4/FD4_CE100_1_0x182/RrCoolantflow ==
  RrCoolantflow : Inport
  Data Type Conversion : DataTypeConversion  OutDataTypeStr=uint8  RndMeth=Round
  convert_out : FVT_lib/hal/convert_out  gain=0.25  offset=0
  CAN4_Rr_Coolantflow : Outport
  wires:
  Data Type Conversion/1 -> CAN4_Rr_Coolantflow/1
  convert_out/1 -> Data Type Conversion/1
  RrCoolantflow/1 -> convert_out/1

== system halout/HAL_OUT/CAN4/FD4_CE100_1_0x182/RrCoolanttemp ==
  RrCoolanttemp : Inport
  Data Type Conversion : DataTypeConversion  OutDataTypeStr=uint16  RndMeth=Round
  convert_out : FVT_lib/hal/convert_out  gain=1  offset=-40
  CAN4_Rr_Coolanttemp : Outport
  wires:
  Data Type Conversion/1 -> CAN4_Rr_Coolanttemp/1
  convert_out/1 -> Data Type Conversion/1
  RrCoolanttemp/1 -> convert_out/1

== system halout/HAL_OUT/CAN4/FD4_CE100_1_0x182/sigAirIntenZon1St ==
  sigAirIntenZon1St : Inport
  Data Type Conversion : DataTypeConversion  OutDataTypeStr=uint8  RndMeth=Round
  CAN4_sigAirIntenZon1St : Outport
  wires:
  Data Type Conversion/1 -> CAN4_sigAirIntenZon1St/1
  sigAirIntenZon1St/1 -> Data Type Conversion/1

== system halout/HAL_OUT/CAN4/FD4_CE100_1_0x182/sigAirIntenZon3St ==
  sigAirIntenZon3St : Inport
  Data Type Conversion : DataTypeConversion  OutDataTypeStr=uint8  RndMeth=Round
  CAN4_sigAirIntenZon3St : Outport
  wires:
  Data Type Conversion/1 -> CAN4_sigAirIntenZon3St/1
  sigAirIntenZon3St/1 -> Data Type Conversion/1

== system halout/HAL_OUT/CAN4/FD4_CE100_1_0x182/sigAmbAirT ==
  sigAmbAirT : Inport
  Data Type Conversion : DataTypeConversion  OutDataTypeStr=uint8  RndMeth=Round
  convert_out : FVT_lib/hal/convert_out  gain=0.5  offset=-40
  CAN4_sigAmbAirT : Outport
  wires:
  Data Type Conversion/1 -> CAN4_sigAmbAirT/1
  convert_out/1 -> Data Type Conversion/1
  sigAmbAirT/1 -> convert_out/1

== system halout/HAL_OUT/CAN4/FD4_CE100_1_0x182/sigCbnAirT ==
  sigCbnAirT : Inport
  Data Type Conversion : DataTypeConversion  OutDataTypeStr=uint8  RndMeth=Round
  convert_out : FVT_lib/hal/convert_out  gain=0.5  offset=-40
  CAN4_sigCbnAirT : Outport
  wires:
  Data Type Conversion/1 -> CAN4_sigCbnAirT/1
  convert_out/1 -> Data Type Conversion/1
  sigCbnAirT/1 -> convert_out/1

== system halout/HAL_OUT/CAN4/FD4_CE100_1_0x182/sigCbnPTCPwrAct ==
  sigCbnPTCPwrAct : Inport
  Data Type Conversion : DataTypeConversion  OutDataTypeStr=uint8  RndMeth=Round
  convert_out : FVT_lib/hal/convert_out  gain=50  offset=0
  CAN4_sigCbnPTCPwrAct : Outport
  wires:
  Data Type Conversion/1 -> CAN4_sigCbnPTCPwrAct/1
  convert_out/1 -> Data Type Conversion/1
  sigCbnPTCPwrAct/1 -> convert_out/1

== system halout/HAL_OUT/CAN4/FD4_CE100_1_0x182/sigCbnSolarLeft ==
  sigCbnSolarLeft : Inport
  Data Type Conversion : DataTypeConversion  OutDataTypeStr=uint8  RndMeth=Round
  convert_out : FVT_lib/hal/convert_out  gain=5  offset=0
  CAN4_sigCbnSolarLeft : Outport
  wires:
  Data Type Conversion/1 -> CAN4_sigCbnSolarLeft/1
  convert_out/1 -> Data Type Conversion/1
  sigCbnSolarLeft/1 -> convert_out/1

== system halout/HAL_OUT/CAN4/FD4_CE100_1_0x182/sigCbnSolarRight ==
  sigCbnSolarRight : Inport
  Data Type Conversion : DataTypeConversion  OutDataTypeStr=uint8  RndMeth=Round
  convert_out : FVT_lib/hal/convert_out  gain=5  offset=0
  CAN4_sigCbnSolarRight : Outport
  wires:
  Data Type Conversion/1 -> CAN4_sigCbnSolarRight/1
  convert_out/1 -> Data Type Conversion/1
  sigCbnSolarRight/1 -> convert_out/1

== system halout/HAL_OUT/CAN4/FD4_CE100_1_0x182/sigClmtCmprPwrAct ==
  sigClmtCmprPwrAct : Inport
  Data Type Conversion : DataTypeConversion  OutDataTypeStr=uint8  RndMeth=Round
  convert_out : FVT_lib/hal/convert_out  gain=50  offset=0
  CAN4_sigClmtCmprPwrAct : Outport
  wires:
  Data Type Conversion/1 -> CAN4_sigClmtCmprPwrAct/1
  convert_out/1 -> Data Type Conversion/1
  sigClmtCmprPwrAct/1 -> convert_out/1

== system halout/HAL_OUT/CAN4/FD4_CE100_1_0x182/sigClntTHvBattOut ==
  sigClntTHvBattOut : Inport
  Data Type Conversion : DataTypeConversion  OutDataTypeStr=uint8  RndMeth=Round
  convert_out : FVT_lib/hal/convert_out  gain=0.5  offset=-40
  CAN4_sigClntTHvBattOut : Outport
  wires:
  Data Type Conversion/1 -> CAN4_sigClntTHvBattOut/1
  convert_out/1 -> Data Type Conversion/1
  sigClntTHvBattOut/1 -> convert_out/1

== system halout/HAL_OUT/CAN4/FD4_CE100_1_0x182/sigDfrstSt ==
  sigDfrstSt : Inport
  Data Type Conversion : DataTypeConversion  OutDataTypeStr=uint8  RndMeth=Round
  CAN4_sigDfrstSt : Outport
  wires:
  Data Type Conversion/1 -> CAN4_sigDfrstSt/1
  sigDfrstSt/1 -> Data Type Conversion/1

== system halout/HAL_OUT/CAN4/FD4_CE100_1_0x182/sigHvacSt ==
  sigHvacSt : Inport
  Data Type Conversion : DataTypeConversion  OutDataTypeStr=uint8  RndMeth=Round
  CAN4_sigHvacSt : Outport
  wires:
  Data Type Conversion/1 -> CAN4_sigHvacSt/1
  sigHvacSt/1 -> Data Type Conversion/1

== system halout/HAL_OUT/CAN4/FD4_CE100_1_0x182/sigRecircSt ==
  sigRecircSt : Inport
  Data Type Conversion : DataTypeConversion  OutDataTypeStr=uint8  RndMeth=Round
  CAN4_sigRecircSt : Outport
  wires:
  Data Type Conversion/1 -> CAN4_sigRecircSt/1
  sigRecircSt/1 -> Data Type Conversion/1

== system halout/HAL_OUT/CAN4/FD4_CE100_1_0x182/sigSetTempZon1St ==
  sigSetTempZon1St : Inport
  Data Type Conversion : DataTypeConversion  OutDataTypeStr=uint8  RndMeth=Round
  convert_out : FVT_lib/hal/convert_out  gain=0.5  offset=17
  CAN4_sigSetTempZon1St : Outport
  wires:
  Data Type Conversion/1 -> CAN4_sigSetTempZon1St/1
  convert_out/1 -> Data Type Conversion/1
  sigSetTempZon1St/1 -> convert_out/1

== system halout/HAL_OUT/CAN4/FD4_CE100_1_0x182/sigSetTempZon2St ==
  sigSetTempZon2St : Inport
  Data Type Conversion : DataTypeConversion  OutDataTypeStr=uint8  RndMeth=Round
  convert_out : FVT_lib/hal/convert_out  gain=0.5  offset=17
  CAN4_sigSetTempZon2St : Outport
  wires:
  Data Type Conversion/1 -> CAN4_sigSetTempZon2St/1
  convert_out/1 -> Data Type Conversion/1
  sigSetTempZon2St/1 -> convert_out/1

== system halout/HAL_OUT/CAN4/FD4_CE100_1_0x182/sigSetTempZon3St ==
  sigSetTempZon3St : Inport
  Data Type Conversion : DataTypeConversion  OutDataTypeStr=uint8  RndMeth=Round
  convert_out : FVT_lib/hal/convert_out  gain=0.5  offset=17
  CAN4_sigSetTempZon3St : Outport
  wires:
  Data Type Conversion/1 -> CAN4_sigSetTempZon3St/1
  convert_out/1 -> Data Type Conversion/1
  sigSetTempZon3St/1 -> convert_out/1

== system halout/HAL_OUT/CAN4/FD4_CE100_1_0x182/sigWindDirZon1St ==
  sigWindDirZon1St : Inport
  Data Type Conversion : DataTypeConversion  OutDataTypeStr=uint8  RndMeth=Round
  CAN4_sigWindDirZon1St : Outport
  wires:
  Data Type Conversion/1 -> CAN4_sigWindDirZon1St/1
  sigWindDirZon1St/1 -> Data Type Conversion/1

== system halout/HAL_OUT/CAN4/FD4_CE100_1_0x182/sigWindDirZon3St ==
  sigWindDirZon3St : Inport
  Data Type Conversion : DataTypeConversion  OutDataTypeStr=uint8  RndMeth=Round
  CAN4_sigWindDirZon3St : Outport
  wires:
  Data Type Conversion/1 -> CAN4_sigWindDirZon3St/1
  sigWindDirZon3St/1 -> Data Type Conversion/1

== system halout/HAL_OUT/CAN4/FD4_CE100_3_0x201/FDCBCMBBuzzerCmd ==
  FDCBCMBBuzzerCmd : Inport
  Data Type Conversion : DataTypeConversion  OutDataTypeStr=uint8  RndMeth=Round
  CAN4_FDC_BCM_BBuzzer_Cmd : Outport
  wires:
  Data Type Conversion/1 -> CAN4_FDC_BCM_BBuzzer_Cmd/1
  FDCBCMBBuzzerCmd/1 -> Data Type Conversion/1

== system halout/HAL_OUT/CAN4/FD4_CE100_3_0x201/FDCBCMBBuzzeroutCmd ==
  FDCBCMBBuzzeroutCmd : Inport
  Data Type Conversion : DataTypeConversion  OutDataTypeStr=uint8  RndMeth=Round
  CAN4_FDC_BCM_BBuzzerout_Cmd : Outport
  wires:
  Data Type Conversion/1 -> CAN4_FDC_BCM_BBuzzerout_Cmd/1
  FDCBCMBBuzzeroutCmd/1 -> Data Type Conversion/1

== system halout/HAL_OUT/CAN4/FD4_CE100_3_0x201/FDCBCMEmExitLightCmd ==
  FDCBCMEmExitLightCmd : Inport
  Data Type Conversion : DataTypeConversion  OutDataTypeStr=uint8  RndMeth=Round
  CAN4_FDC_BCM_EmExitLight_Cmd : Outport
  wires:
  Data Type Conversion/1 -> CAN4_FDC_BCM_EmExitLight_Cmd/1
  FDCBCMEmExitLightCmd/1 -> Data Type Conversion/1

== system halout/HAL_OUT/CAN4/FD4_CE100_3_0x201/FDCBCMFrAtmoLampCmd ==
  FDCBCMFrAtmoLampCmd : Inport
  Data Type Conversion : DataTypeConversion  OutDataTypeStr=uint8  RndMeth=Round
  CAN4_FDC_BCM_FrAtmoLamp_Cmd : Outport
  wires:
  Data Type Conversion/1 -> CAN4_FDC_BCM_FrAtmoLamp_Cmd/1
  FDCBCMFrAtmoLampCmd/1 -> Data Type Conversion/1

== system halout/HAL_OUT/CAN4/FD4_CE100_3_0x201/FDCBCMFrRmLampBrightCmd ==
  FDCBCMFrRmLampBrightCmd : Inport
  Data Type Conversion : DataTypeConversion  OutDataTypeStr=uint8  RndMeth=Round
  CAN4_FDC_BCM_FrRmLampBright_Cmd : Outport
  wires:
  Data Type Conversion/1 -> CAN4_FDC_BCM_FrRmLampBright_Cmd/1
  FDCBCMFrRmLampBrightCmd/1 -> Data Type Conversion/1

== system halout/HAL_OUT/CAN4/FD4_CE100_3_0x201/FDCBCMFrRoomlampCmd ==
  FDCBCMFrRoomlampCmd : Inport
  Data Type Conversion : DataTypeConversion  OutDataTypeStr=uint8  RndMeth=Round
  CAN4_FDC_BCM_FrRoomlamp_Cmd : Outport
  wires:
  Data Type Conversion/1 -> CAN4_FDC_BCM_FrRoomlamp_Cmd/1
  FDCBCMFrRoomlampCmd/1 -> Data Type Conversion/1

== system halout/HAL_OUT/CAN4/FD4_CE100_3_0x201/FDCBCMIBuzzerReqSta ==
  FDCBCMIBuzzerReqSta : Inport
  Data Type Conversion : DataTypeConversion  OutDataTypeStr=uint8  RndMeth=Round
  CAN4_FDC_BCM_IBuzzerReq_Sta : Outport
  wires:
  Data Type Conversion/1 -> CAN4_FDC_BCM_IBuzzerReq_Sta/1
  FDCBCMIBuzzerReqSta/1 -> Data Type Conversion/1

== system halout/HAL_OUT/CAN4/FD4_CE100_3_0x201/FDCBCMLSMLPCmd ==
  FDCBCMLSMLPCmd : Inport
  Data Type Conversion : DataTypeConversion  OutDataTypeStr=uint8  RndMeth=Round
  CAN4_FDC_BCM_LSMLP_Cmd : Outport
  wires:
  Data Type Conversion/1 -> CAN4_FDC_BCM_LSMLP_Cmd/1
  FDCBCMLSMLPCmd/1 -> Data Type Conversion/1

== system halout/HAL_OUT/CAN4/FD4_CE100_3_0x201/FDCBCMLTgateRelCmd ==
  FDCBCMLTgateRelCmd : Inport
  Data Type Conversion : DataTypeConversion  OutDataTypeStr=uint8  RndMeth=Round
  CAN4_FDC_BCM_LTgateRel_Cmd : Outport
  wires:
  Data Type Conversion/1 -> CAN4_FDC_BCM_LTgateRel_Cmd/1
  FDCBCMLTgateRelCmd/1 -> Data Type Conversion/1

== system halout/HAL_OUT/CAN4/FD4_CE100_3_0x201/FDCBCMRSMLPCmd ==
  FDCBCMRSMLPCmd : Inport
  Data Type Conversion : DataTypeConversion  OutDataTypeStr=uint8  RndMeth=Round
  CAN4_FDC_BCM_RSMLP_Cmd : Outport
  wires:
  Data Type Conversion/1 -> CAN4_FDC_BCM_RSMLP_Cmd/1
  FDCBCMRSMLPCmd/1 -> Data Type Conversion/1

== system halout/HAL_OUT/CAN4/FD4_CE100_3_0x201/FDCBCMRTgateRelCmd ==
  FDCBCMRTgateRelCmd : Inport
  Data Type Conversion : DataTypeConversion  OutDataTypeStr=uint8  RndMeth=Round
  CAN4_FDC_BCM_RTgateRel_Cmd : Outport
  wires:
  Data Type Conversion/1 -> CAN4_FDC_BCM_RTgateRel_Cmd/1
  FDCBCMRTgateRelCmd/1 -> Data Type Conversion/1

== system halout/HAL_OUT/CAN4/FD4_CE100_3_0x201/FDCBCMRevBuzzeroutCmd ==
  FDCBCMRevBuzzeroutCmd : Inport
  Data Type Conversion : DataTypeConversion  OutDataTypeStr=uint8  RndMeth=Round
  CAN4_FDC_BCM_RevBuzzerout_Cmd : Outport
  wires:
  Data Type Conversion/1 -> CAN4_FDC_BCM_RevBuzzerout_Cmd/1
  FDCBCMRevBuzzeroutCmd/1 -> Data Type Conversion/1

== system halout/HAL_OUT/CAN4/FD4_CE100_3_0x201/FDCBCMRrAtmoLampCmd ==
  FDCBCMRrAtmoLampCmd : Inport
  Data Type Conversion : DataTypeConversion  OutDataTypeStr=uint8  RndMeth=Round
  CAN4_FDC_BCM_RrAtmoLamp_Cmd : Outport
  wires:
  Data Type Conversion/1 -> CAN4_FDC_BCM_RrAtmoLamp_Cmd/1
  FDCBCMRrAtmoLampCmd/1 -> Data Type Conversion/1

== system halout/HAL_OUT/CAN4/FD4_CE100_3_0x201/FDCBCMRrRmLampBrightCmd ==
  FDCBCMRrRmLampBrightCmd : Inport
  Data Type Conversion : DataTypeConversion  OutDataTypeStr=uint8  RndMeth=Round
  CAN4_FDC_BCM_RrRmLampBright_Cmd : Outport
  wires:
  Data Type Conversion/1 -> CAN4_FDC_BCM_RrRmLampBright_Cmd/1
  FDCBCMRrRmLampBrightCmd/1 -> Data Type Conversion/1

== system halout/HAL_OUT/CAN4/FD4_CE100_3_0x201/FDCBCMRrRoomlampCmd ==
  FDCBCMRrRoomlampCmd : Inport
  Data Type Conversion : DataTypeConversion  OutDataTypeStr=uint8  RndMeth=Round
  CAN4_FDC_BCM_RrRoomlamp_Cmd : Outport
  wires:
  Data Type Conversion/1 -> CAN4_FDC_BCM_RrRoomlamp_Cmd/1
  FDCBCMRrRoomlampCmd/1 -> Data Type Conversion/1

== system halout/HAL_OUT/CAN4/FD4_CE100_3_0x201/FDCBCMSTurnLpLeftCmd ==
  FDCBCMSTurnLpLeftCmd : Inport
  Data Type Conversion : DataTypeConversion  OutDataTypeStr=uint8  RndMeth=Round
  CAN4_FDC_BCM_STurnLpLeft_Cmd : Outport
  wires:
  Data Type Conversion/1 -> CAN4_FDC_BCM_STurnLpLeft_Cmd/1
  FDCBCMSTurnLpLeftCmd/1 -> Data Type Conversion/1

== system halout/HAL_OUT/CAN4/FD4_CE100_3_0x201/FDCBCMSTurnLpRightCmd ==
  FDCBCMSTurnLpRightCmd : Inport
  Data Type Conversion : DataTypeConversion  OutDataTypeStr=uint8  RndMeth=Round
  CAN4_FDC_BCM_STurnLpRight_Cmd : Outport
  wires:
  Data Type Conversion/1 -> CAN4_FDC_BCM_STurnLpRight_Cmd/1
  FDCBCMSTurnLpRightCmd/1 -> Data Type Conversion/1

== system halout/HAL_OUT/CAN4/FD4_CE100_3_0x201/FDCBCMTgateHDSWLSta ==
  FDCBCMTgateHDSWLSta : Inport
  Data Type Conversion : DataTypeConversion  OutDataTypeStr=uint8  RndMeth=Round
  CAN4_FDC_BCM_TgateHDSWL_Sta : Outport
  wires:
  Data Type Conversion/1 -> CAN4_FDC_BCM_TgateHDSWL_Sta/1
  FDCBCMTgateHDSWLSta/1 -> Data Type Conversion/1

== system halout/HAL_OUT/CAN4/FD4_CE100_3_0x201/FDCBCMTgateHDSWRSta ==
  FDCBCMTgateHDSWRSta : Inport
  Data Type Conversion : DataTypeConversion  OutDataTypeStr=uint8  RndMeth=Round
  CAN4_FDC_BCM_TgateHDSWR_Sta : Outport
  wires:
  Data Type Conversion/1 -> CAN4_FDC_BCM_TgateHDSWR_Sta/1
  FDCBCMTgateHDSWRSta/1 -> Data Type Conversion/1

== system halout/HAL_OUT/CAN4/FD4_CE100_3_0x201/FDCBCMTgateSWLSta ==
  FDCBCMTgateSWLSta : Inport
  Data Type Conversion : DataTypeConversion  OutDataTypeStr=uint8  RndMeth=Round
  CAN4_FDC_BCM_TgateSWL_Sta : Outport
  wires:
  Data Type Conversion/1 -> CAN4_FDC_BCM_TgateSWL_Sta/1
  FDCBCMTgateSWLSta/1 -> Data Type Conversion/1

== system halout/HAL_OUT/CAN4/FD4_CE100_3_0x201/FDCBCMTgateSWRSta ==
  FDCBCMTgateSWRSta : Inport
  Data Type Conversion : DataTypeConversion  OutDataTypeStr=uint8  RndMeth=Round
  CAN4_FDC_BCM_TgateSWR_Sta : Outport
  wires:
  Data Type Conversion/1 -> CAN4_FDC_BCM_TgateSWR_Sta/1
  FDCBCMTgateSWRSta/1 -> Data Type Conversion/1

== system halout/HAL_OUT/CAN4/FD4_CE100_3_0x201/FDCBCMTurnLpLActiveCmd ==
  FDCBCMTurnLpLActiveCmd : Inport
  Data Type Conversion : DataTypeConversion  OutDataTypeStr=uint8  RndMeth=Round
  CAN4_FDC_BCM_TurnLpLActive_Cmd : Outport
  wires:
  Data Type Conversion/1 -> CAN4_FDC_BCM_TurnLpLActive_Cmd/1
  FDCBCMTurnLpLActiveCmd/1 -> Data Type Conversion/1

== system halout/HAL_OUT/CAN4/FD4_CE100_3_0x201/FDCBCMTurnLpRActiveCmd ==
  FDCBCMTurnLpRActiveCmd : Inport
  Data Type Conversion : DataTypeConversion  OutDataTypeStr=uint8  RndMeth=Round
  CAN4_FDC_BCM_TurnLpRActive_Cmd : Outport
  wires:
  Data Type Conversion/1 -> CAN4_FDC_BCM_TurnLpRActive_Cmd/1
  FDCBCMTurnLpRActiveCmd/1 -> Data Type Conversion/1

== system halout/HAL_OUT/CAN4/FD4_CE100_3_0x201/FDCBCMinnerBuzzerCmd ==
  FDCBCMinnerBuzzerCmd : Inport
  Data Type Conversion : DataTypeConversion  OutDataTypeStr=uint8  RndMeth=Round
  CAN4_FDC_BCM_innerBuzzer_Cmd : Outport
  wires:
  Data Type Conversion/1 -> CAN4_FDC_BCM_innerBuzzer_Cmd/1
  FDCBCMinnerBuzzerCmd/1 -> Data Type Conversion/1

== system halout/HAL_OUT/CAN4/FD4_CE200_0_0x217/AmbLightBreath1 ==
  AmbLightBreath1 : Inport
  Data Type Conversion : DataTypeConversion  OutDataTypeStr=uint8  RndMeth=Round
  CAN4_AmbLightBreath1 : Outport
  wires:
  Data Type Conversion/1 -> CAN4_AmbLightBreath1/1
  AmbLightBreath1/1 -> Data Type Conversion/1

== system halout/HAL_OUT/CAN4/FD4_CE200_0_0x217/AmbLightBreath2 ==
  AmbLightBreath2 : Inport
  Data Type Conversion : DataTypeConversion  OutDataTypeStr=uint8  RndMeth=Round
  CAN4_AmbLightBreath2 : Outport
  wires:
  Data Type Conversion/1 -> CAN4_AmbLightBreath2/1
  AmbLightBreath2/1 -> Data Type Conversion/1

== system halout/HAL_OUT/CAN4/FD4_CE200_0_0x217/AmbLightBreath3 ==
  AmbLightBreath3 : Inport
  Data Type Conversion : DataTypeConversion  OutDataTypeStr=uint8  RndMeth=Round
  CAN4_AmbLightBreath3 : Outport
  wires:
  Data Type Conversion/1 -> CAN4_AmbLightBreath3/1
  AmbLightBreath3/1 -> Data Type Conversion/1

== system halout/HAL_OUT/CAN4/FD4_CE200_0_0x217/AmbLightBreath4 ==
  AmbLightBreath4 : Inport
  Data Type Conversion : DataTypeConversion  OutDataTypeStr=uint8  RndMeth=Round
  CAN4_AmbLightBreath4 : Outport
  wires:
  Data Type Conversion/1 -> CAN4_AmbLightBreath4/1
  AmbLightBreath4/1 -> Data Type Conversion/1

== system halout/HAL_OUT/CAN4/FD4_CE200_0_0x217/AmbLightBreath5 ==
  AmbLightBreath5 : Inport
  Data Type Conversion : DataTypeConversion  OutDataTypeStr=uint8  RndMeth=Round
  CAN4_AmbLightBreath5 : Outport
  wires:
  Data Type Conversion/1 -> CAN4_AmbLightBreath5/1
  AmbLightBreath5/1 -> Data Type Conversion/1

== system halout/HAL_OUT/CAN4/FD4_CE200_0_0x217/AmbLightBreath6 ==
  AmbLightBreath6 : Inport
  Data Type Conversion : DataTypeConversion  OutDataTypeStr=uint8  RndMeth=Round
  CAN4_AmbLightBreath6 : Outport
  wires:
  Data Type Conversion/1 -> CAN4_AmbLightBreath6/1
  AmbLightBreath6/1 -> Data Type Conversion/1

== system halout/HAL_OUT/CAN4/FD4_CE200_0_0x217/AmbLightBrightness1 ==
  AmbLightBrightness1 : Inport
  Data Type Conversion : DataTypeConversion  OutDataTypeStr=uint8  RndMeth=Round
  CAN4_AmbLightBrightness1 : Outport
  wires:
  Data Type Conversion/1 -> CAN4_AmbLightBrightness1/1
  AmbLightBrightness1/1 -> Data Type Conversion/1

== system halout/HAL_OUT/CAN4/FD4_CE200_0_0x217/AmbLightBrightness2 ==
  AmbLightBrightness2 : Inport
  Data Type Conversion : DataTypeConversion  OutDataTypeStr=uint8  RndMeth=Round
  CAN4_AmbLightBrightness2 : Outport
  wires:
  Data Type Conversion/1 -> CAN4_AmbLightBrightness2/1
  AmbLightBrightness2/1 -> Data Type Conversion/1

== system halout/HAL_OUT/CAN4/FD4_CE200_0_0x217/AmbLightBrightness3 ==
  AmbLightBrightness3 : Inport
  Data Type Conversion : DataTypeConversion  OutDataTypeStr=uint8  RndMeth=Round
  CAN4_AmbLightBrightness3 : Outport
  wires:
  Data Type Conversion/1 -> CAN4_AmbLightBrightness3/1
  AmbLightBrightness3/1 -> Data Type Conversion/1

== system halout/HAL_OUT/CAN4/FD4_CE200_0_0x217/AmbLightBrightness4 ==
  AmbLightBrightness4 : Inport
  Data Type Conversion : DataTypeConversion  OutDataTypeStr=uint8  RndMeth=Round
  CAN4_AmbLightBrightness4 : Outport
  wires:
  Data Type Conversion/1 -> CAN4_AmbLightBrightness4/1
  AmbLightBrightness4/1 -> Data Type Conversion/1

== system halout/HAL_OUT/CAN4/FD4_CE200_0_0x217/AmbLightBrightness5 ==
  AmbLightBrightness5 : Inport
  Data Type Conversion : DataTypeConversion  OutDataTypeStr=uint8  RndMeth=Round
  CAN4_AmbLightBrightness5 : Outport
  wires:
  Data Type Conversion/1 -> CAN4_AmbLightBrightness5/1
  AmbLightBrightness5/1 -> Data Type Conversion/1

== system halout/HAL_OUT/CAN4/FD4_CE200_0_0x217/AmbLightBrightness6 ==
  AmbLightBrightness6 : Inport
  Data Type Conversion : DataTypeConversion  OutDataTypeStr=uint8  RndMeth=Round
  CAN4_AmbLightBrightness6 : Outport
  wires:
  Data Type Conversion/1 -> CAN4_AmbLightBrightness6/1
  AmbLightBrightness6/1 -> Data Type Conversion/1

== system halout/HAL_OUT/CAN4/FD4_CE200_0_0x217/AmbLightColor1 ==
  AmbLightColor1 : Inport
  Data Type Conversion : DataTypeConversion  OutDataTypeStr=uint8  RndMeth=Round
  CAN4_AmbLightColor1 : Outport
  wires:
  Data Type Conversion/1 -> CAN4_AmbLightColor1/1
  AmbLightColor1/1 -> Data Type Conversion/1

== system halout/HAL_OUT/CAN4/FD4_CE200_0_0x217/AmbLightColor2 ==
  AmbLightColor2 : Inport
  Data Type Conversion : DataTypeConversion  OutDataTypeStr=uint8  RndMeth=Round
  CAN4_AmbLightColor2 : Outport
  wires:
  Data Type Conversion/1 -> CAN4_AmbLightColor2/1
  AmbLightColor2/1 -> Data Type Conversion/1

== system halout/HAL_OUT/CAN4/FD4_CE200_0_0x217/AmbLightColor3 ==
  AmbLightColor3 : Inport
  Data Type Conversion : DataTypeConversion  OutDataTypeStr=uint8  RndMeth=Round
  CAN4_AmbLightColor3 : Outport
  wires:
  Data Type Conversion/1 -> CAN4_AmbLightColor3/1
  AmbLightColor3/1 -> Data Type Conversion/1
